simulink model "SSi_liftup"  (R2024b)
settings: Solver=ode1  StartTime=0.0  StopTime=20  FixedStep=0.002  RelTol=1e-3  EnableMultiTasking=on
PostLoadFcn:
  | qc_set_target_type(getConfigSet(bdroot, 'QUARC Default Target Configuration'));
undefined symbols (not defined in the file): A_sw, Aobs, Aobs_d, B_sw, Bobs, Bobs_d, c_star, C_sw, Cobs, Cobs_d, DiscIntNeverNeededParam, HIL, init_cond_lift, K5, K_p2, K_phase1_int, K_phase1_pd, P_end, T1_val, t_p1, t_p2, Ts, u_p1, u_p2, ud_neg, ud_pos, V_sat, x_p1, x_p2
libraries: quarc_library x4
settings Model: SimulationMode=external  ExtModeTrigDuration=5000  Creator=pmartin  LastModifiedBy=natha
settings SolverCC: AlgebraicLoopSolver=TrustRegion  PositivePriorityOrder=on
settings DataIOCC: LimitDataPoints=on  SaveFormat=Array  SignalLoggingSaveFormat=ModelDataLogs  ReturnWorkspaceOutputs=off
settings OptimizationCC: ExpressionDepthLimit=2147483647  InitFltsAndDblsToZero=on
settings DebuggingCC: SaveWithParameterizedLinksMsg=none  UnderspecifiedInitializationDetection=Classic  MergeDetectMultiDrivingBlocksExec=none  SolverPrmCheckMsg=warning  MultiTaskDSMMsg=warning  MultiTaskCondExecSysMsg=none  FcnCallInpInsideContextMsg=warning  UnconnectedInputMsg=warning  UnconnectedOutputMsg=warning  UnconnectedLineMsg=warning  StateNameClashWarn=warning  SFUnexpectedBacktrackingDiag=warning  SFNoUnconditionalDefaultTransitionDiag=warning  SFExecutionAtInitializationDiag=none  ArithmeticOperatorsInVariantConditions=warning
settings ModelReferenceCC: PropagateSignalLabelsOutOfModel=off
settings SFSimCC: SimUseLocalCustomCode=off  CustomCodeUndefinedFunction=UseInterfaceOnly
settings RTWCC: RTWUseLocalCustomCode=off  Toolchain=QUARC win64 | nmake (64-bit Windows)  BuildConfiguration=Faster Runs  GPUComputeCapability=3.5
settings CodeAppCC: StateflowObjectComments=on
settings GRTTargetCC: TargetLangStandard=C89/C90 (ANSI)
settings ConfigComp: CovMetricSettings=dw  CovSaveCumulativeToWorkspaceVar=on  CovSaveSingleToWorkspaceVar=on  CovExternalEMLEnable=off

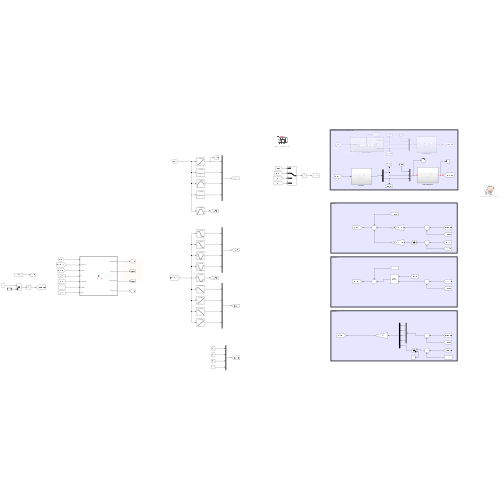
[thumbnail: Simulink's stored preview of the top-level diagram]
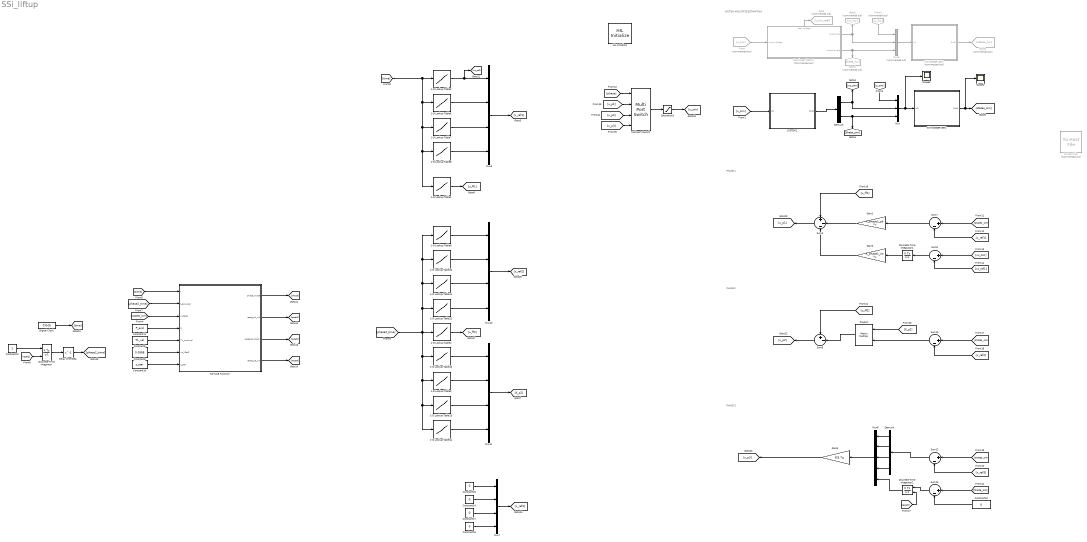
== system SSi_liftup ==
  note: PHASE 1
  note: MOTOR AND STATE ESTIMATION
  note: PHASE 2
  note: PHASE 3
  1-D Lookup Table1 : Lookup_n-D  NumberOfTableDimensions=1  BreakpointsForDimension1=t_p1  Table=u_p1  InternalRulePriority=Speed  RndMeth=Simplest
  1-D Lookup Table10 : Lookup_n-D  NumberOfTableDimensions=1  BreakpointsForDimension1=t_p2  Table=x_p2(:,2)  InternalRulePriority=Speed  RndMeth=Simplest
  1-D Lookup Table11 : Lookup_n-D  NumberOfTableDimensions=1  BreakpointsForDimension1=t_p2  Table=x_p2(:,3)  InternalRulePriority=Speed  RndMeth=Simplest
  1-D Lookup Table12 : Lookup_n-D  NumberOfTableDimensions=1  BreakpointsForDimension1=t_p2  Table=x_p2(:,4)  InternalRulePriority=Speed  RndMeth=Simplest
  1-D Lookup Table13 : Lookup_n-D  NumberOfTableDimensions=1  BreakpointsForDimension1=t_p2  Table=K_p2(:,3)  InternalRulePriority=Speed  RndMeth=Simplest
  1-D Lookup Table14 : Lookup_n-D  NumberOfTableDimensions=1  BreakpointsForDimension1=t_p2  Table=K_p2(:,4)  InternalRulePriority=Speed  RndMeth=Simplest
  1-D Lookup Table15 : Lookup_n-D  NumberOfTableDimensions=1  BreakpointsForDimension1=t_p2  Table=K_p2(:,1)  InternalRulePriority=Speed  RndMeth=Simplest
  1-D Lookup Table2 : Lookup_n-D  NumberOfTableDimensions=1  BreakpointsForDimension1=t_p1  Table=x_p1(:,1)  InternalRulePriority=Speed  RndMeth=Simplest
  1-D Lookup Table3 : Lookup_n-D  NumberOfTableDimensions=1  BreakpointsForDimension1=t_p2  Table=K_p2(:,2)  InternalRulePriority=Speed  RndMeth=Simplest
  1-D Lookup Table4 : Lookup_n-D  NumberOfTableDimensions=1  BreakpointsForDimension1=t_p2  Table=u_p2  InternalRulePriority=Speed  RndMeth=Simplest
  1-D Lookup Table6 : Lookup_n-D  NumberOfTableDimensions=1  BreakpointsForDimension1=t_p1  Table=x_p1(:,2)  InternalRulePriority=Speed  RndMeth=Simplest
  1-D Lookup Table7 : Lookup_n-D  NumberOfTableDimensions=1  BreakpointsForDimension1=t_p1  Table=x_p1(:,3)  InternalRulePriority=Speed  RndMeth=Simplest
  1-D Lookup Table8 : Lookup_n-D  NumberOfTableDimensions=1  BreakpointsForDimension1=t_p1  Table=x_p1(:,4)  InternalRulePriority=Speed  RndMeth=Simplest
  1-D Lookup Table9 : Lookup_n-D  NumberOfTableDimensions=1  BreakpointsForDimension1=t_p2  Table=x_p2(:,1)  InternalRulePriority=Speed  RndMeth=Simplest
  Constant10 : Constant  Value=c_star
  Constant11 : Constant  Value=P_end
  Constant12 : Constant
  Constant{13..17} (5 alike) : Constant  Value=0
  Constant8 : Constant  Value=T1_val
  Constant9 : Constant  Value=0.0568
  Delay One Step : Delay  DelayLength=1
  Demux3 : Demux  Outputs=2
  Demux4 : Demux
  Digital Clock : DigitalClock  SampleTime=Ts
  Discrete-Time Integrator : DiscreteIntegrator  ExternalReset=rising  SampleTime=-1  ICPrevOutput=DiscIntNeverNeededParam  ICPrevScaledInput=DiscIntNeverNeededParam
  Discrete-Time Integrator1 : DiscreteIntegrator  SampleTime=-1  ICPrevOutput=DiscIntNeverNeededParam  ICPrevScaledInput=DiscIntNeverNeededParam
  Discrete-Time Integrator2 : DiscreteIntegrator  ExternalReset=rising  SampleTime=-1  ICPrevOutput=DiscIntNeverNeededParam  ICPrevScaledInput=DiscIntNeverNeededParam
  From : From  Commented=on  GotoTag=u_hw
  From3 : From  Commented=on  GotoTag=u_hw
  Gain2 : Gain  Gain=K_phase1_pd  Multiplication=Matrix(K*u)
  Gain3 : Gain  Gain=K_phase1_int  Multiplication=Matrix(K*u)
  Gain5 : Gain  Gain=K5  Multiplication=Matrix(K*u)
  Goto : Goto  Commented=on  GotoTag=u_hw_real
  Goto1 : Goto  Commented=on  GotoTag=theta_hw
  Goto2 : Goto  Commented=on  GotoTag=xc_hw
  Goto8 : Goto  Commented=on  GotoTag=states_hw
  HIL Initialize : quarc_library/Data Acquisition/Generic/Configuration/HIL Initialize  object_name=HIL-1  board_type=---- Quanser ----  board_number=0  board_options=d0=digital;d1=digital;led=auto;update_rate=normal  exclusive=off  active=off  hardware_clocks=[0:2]  clock_modes=[]  initial_clock_frequencies=[]  set_clock_params_at_start=off  set_clock_params_at_switch_in=off  set_clock_frequencies_at_start=off  set_clock_frequencies_at_switch_in=off  analog_input_channels=[0:1]  analog_input_configurations=[]  analog_input_maximums=10  analog_input_minimums=-10  set_analog_input_params_at_start=on  set_analog_input_params_at_switch_in=off  analog_output_channels=[0:1]  analog_output_maximums=10  analog_output_minimums=-10  initial_analog_outputs=[0]  final_analog_outputs=[0]  watchdog_analog_outputs=0  set_analog_output_params_at_start=on  set_analog_output_params_at_switch_in=off  set_analog_outputs_at_start=on  set_analog_outputs_at_switch_in=off  set_analog_outputs_at_terminate=on  set_analog_outputs_at_switch_out=off  set_analog_outputs_on_watchdog=off  digital_input_channels=[]  digital_output_channels=[0:7]  digital_output_configuration=[]  initial_digital_outputs=[0]  final_digital_outputs=[0]  watchdog_digital_outputs=[0]  set_digital_output_params_at_start=off  set_digital_output_params_at_switch_in=off  set_digital_outputs_at_start=on  set_digital_outputs_at_switch_in=off  set_digital_outputs_at_terminate=on  set_digital_outputs_at_switch_out=off  set_digital_outputs_on_watchdog=off  encoder_channels=[0:1]  quadrature=[4]  encoder_filter_frequency=[]  initial_encoder_counts=[0]  set_encoder_params_at_start=on  set_encoder_params_at_switch_in=off  set_encoder_counts_at_start=on  set_encoder_counts_at_switch_in=off  pwm_channels=[]  pwm_modes=[0]  pwm_frequency=1/0.020  pwm_configuration=[]  pwm_alignment=[]  pwm_polarity=[]  pwm_leading_deadband=[]  pwm_trailing_deadband=[]  initial_pwm_outputs=[0]  final_pwm_outputs=[0]  watchdog_pwm_outputs=[0]  set_pwm_params_at_start=on  set_pwm_params_at_switch_in=off  set_pwm_outputs_at_start=on  set_pwm_outputs_at_switch_in=off  set_pwm_outputs_at_terminate=on  set_pwm_outputs_at_switch_out=off  set_pwm_outputs_on_watchdog=off  other_output_channels=[]  initial_other_outputs=[]  final_other_outputs=[]  watchdog_other_outputs=[]  set_other_outputs_at_start=off  set_other_outputs_at_switch_in=off  set_other_outputs_at_terminate=off  set_other_outputs_at_switch_out=off  set_other_outputs_on_watchdog=off
  HW OBSERVER1 : Subsystem  Commented=on
  MATLAB Function : MATLAB Function  TreatAsAtomicUnit=on
  Multiport Switch : MultiPortSwitch  SaturateOnIntegerOverflow=off  InputSameDT=off
  Mux : Mux  Inputs=3
  Mux{7,9..11} (4 alike) : Mux
  Mux6 : Mux  Commented=on  Inputs=3
  Mux8 : Mux  Inputs=5
  Non-linear Motor1 : Subsystem  Commented=on
      settings: PortSchema="{\"entries\":[{\"content\":{\"sides\":[{\"content\":{\"connectorIds\":[\"In1\"]},\"type\":\"ConnectorPlacement.EquallySpacedRectSide\",\"uuid\":\"8ae262a2-80f5-49ad-9b79-cc35ec5329ff\"},{\"content\":{\"connectorIds\":[\"Out1\",\"Out2\"],\"side\":\"RIGHT\"},\"type\":\"ConnectorPlacement.EquallySpacedRectSide\",\"uuid\":\"cff0d77c-9ae7-4fa2-97d7-b58b6cdbe1a2\"},{\"content\":{\"connectorIds\":[\"Out3\"],\"side\":\"TOP\"},\"type\":\"ConnectorPlacement.EquallySpacedRectSide\",\"uuid\":\"5d4527f6-0b4e-4e3d-a127-4f94b563ffba\"}]},\"type\":\"ConnectorPlacement.EquallySpacedConnector\",\"uuid\":\"e038adc8-37ae-49b9-ae92-fde38d51b088\"}],\"packageUris\":[\"http://schema.mathworks.com/mf0/Connector/R2020b\"],\"version\":\"1.0\"}"
  Product : Product  Multiplication=Matrix(*)
  SYM OBSERVER1 : Subsystem
  SYSTEM1 : Subsystem
  Saturation2 : Saturate  UpperLimit=6  LowerLimit=-6
  Scope2 : Scope
  Scope3 : Scope
  Sum{7..8,10,12..13} (5 alike) : Sum  Inputs=|+-
  Sum3 : Sum  Inputs=+--
  Sum9 : Sum  Inputs=+-|
  To Host File : quarc_library/Sinks/To Host/To Host File  Commented=on  source=Specify via dialog (do not evaluate)  file_name=data_%{date}_%{time}.mat  variable_name=data  decimation=1  sample_time=-1  file_format=MAT-file v.4  options=No header or footer  append=off  final_file_name=data_22-May-2026_21-27-47.mat  encoding=Default  bitrate=0
  wires:
  From/1 -> Non-linear Motor1/1(input voltage)
  [u_sim] -> SYSTEM1/1(In1)
  SYSTEM1/1(Out1) -> Demux3/1
  Non-linear Motor1/3(real voltage) -> Goto/1
  Demux3/1 -> Mux/2, [xc_sim]
  Demux3/2 -> [theta_sim], Mux/3
  Constant8/1 -> MATLAB Function/5(T1_nominal)
  Constant9/1 -> MATLAB Function/6(xc_liftoff)
  Constant10/1 -> MATLAB Function/7(c_star)
  [u_sim] -> Mux/1
  Mux/1 -> Scope3/1, SYM OBSERVER1/1(In1)
  From3/1 -> Mux6/1
  Non-linear Motor1/1(output pos) -> Mux6/2, Goto2/1
  Mux6/1 -> HW OBSERVER1/1(In1)
  Non-linear Motor1/2(output angle) -> Mux6/3, Goto1/1
  HW OBSERVER1/1(Out1) -> Goto8/1
  SYM OBSERVER1/1(Out1) -> Scope2/1, [states_sim]
  [time] -> MATLAB Function/1(t)
  Constant11/1 -> MATLAB Function/4(P)
  Digital Clock/1 -> [time]
  [states_sim] -> MATLAB Function/3(x_state)
  MATLAB Function/1(phase_mode) -> [phase]
  MATLAB Function/2(reset_p1_int) -> [reset1]
  MATLAB Function/3(reset_p2_clock) -> [reset2]
  MATLAB Function/4(reset_p3_int) -> [reset3]
  Constant12/1 -> Discrete-Time Integrator/1
  Discrete-Time Integrator/1 -> Delay One Step/1
  [reset2] -> Discrete-Time Integrator/2
  [phase2_time] -> MATLAB Function/2(t_p2_local)
  1-D Lookup Table1/1 -> [u_ff1]
  1-D Lookup Table4/1 -> [u_ff2]
  [phase] -> Multiport Switch/1
  Multiport Switch/1 -> Saturation2/1
  Sum3/1 -> [u_p1]
  [states_sim] -> Sum7/1
  [x_ref1] -> Sum7/2
  [xc_sim] -> Sum8/1
  [xc_ref1] -> Sum8/2
  Sum8/1 -> Discrete-Time Integrator1/1
  Sum7/1 -> Gain2/1
  Discrete-Time Integrator1/1 -> Gain3/1
  [u_ff1] -> Sum3/1
  Gain2/1 -> Sum3/2
  Gain3/1 -> Sum3/3
  [u_p1] -> Multiport Switch/2
  [u_ff2] -> Sum9/1
  Product/1 -> Sum9/2
  Sum9/1 -> [u_p2]
  Sum10/1 -> Product/2
  [states_sim] -> Sum10/1
  [x_ref2] -> Sum10/2
  Constant13/1 -> Sum13/2
  Gain5/1 -> [u_p3]
  [theta_sim] -> Sum13/1
  Sum13/1 -> Discrete-Time Integrator2/1
  Discrete-Time Integrator2/1 -> Mux8/5
  [states_sim] -> Sum12/1
  [x_ref3] -> Sum12/2
  Constant17/1 -> Mux7/3
  Constant15/1 -> Mux7/1
  Constant16/1 -> Mux7/4
  Constant14/1 -> Mux7/2
  Mux7/1 -> [x_ref3]
  [u_p2] -> Multiport Switch/3
  [u_p3] -> Multiport Switch/4
  Sum12/1 -> Demux4/1
  Demux4/1 -> Mux8/1
  Demux4/2 -> Mux8/2
  Demux4/3 -> Mux8/3
  Demux4/4 -> Mux8/4
  Mux8/1 -> Gain5/1
  [K_p2] -> Product/1
  [reset3] -> Discrete-Time Integrator2/2
  [time] -> 1-D Lookup Table2/1, 1-D Lookup Table6/1, 1-D Lookup Table8/1, 1-D Lookup Table1/1, 1-D Lookup Table7/1
  1-D Lookup Table2/1 -> [xc_ref1], Mux9/1
  1-D Lookup Table6/1 -> Mux9/2
  1-D Lookup Table7/1 -> Mux9/3
  1-D Lookup Table8/1 -> Mux9/4
  Mux9/1 -> [x_ref1]
  1-D Lookup Table11/1 -> Mux10/3
  1-D Lookup Table10/1 -> Mux10/2
  1-D Lookup Table12/1 -> Mux10/4
  1-D Lookup Table9/1 -> Mux10/1
  Mux10/1 -> [x_ref2]
  [phase2_time] -> 1-D Lookup Table14/1, 1-D Lookup Table13/1, 1-D Lookup Table3/1, 1-D Lookup Table15/1, 1-D Lookup Table12/1, 1-D Lookup Table11/1, 1-D Lookup Table10/1, 1-D Lookup Table9/1, 1-D Lookup Table4/1
  1-D Lookup Table13/1 -> Mux11/3
  1-D Lookup Table3/1 -> Mux11/2
  1-D Lookup Table15/1 -> Mux11/1
  Mux11/1 -> [K_p2]
  1-D Lookup Table14/1 -> Mux11/4
  Delay One Step/1 -> [phase2_time]
  Saturation2/1 -> [u_sim]

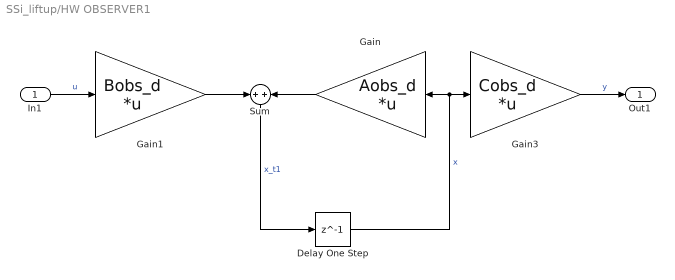
== system SSi_liftup/HW OBSERVER1 ==
  In1 : Inport
  Delay One Step : Delay  DelayLength=1
  Gain : Gain  Gain=Aobs_d  Multiplication=Matrix(K*u)
  Gain1 : Gain  Gain=Bobs_d  Multiplication=Matrix(K*u)
  Gain3 : Gain  Gain=Cobs_d  Multiplication=Matrix(K*u)
  Sum : Sum
  Out1 : Outport
  wires:
  In1/1 -> Gain1/1  "u"
  Gain/1 -> Sum/2
  Gain1/1 -> Sum/1
  Delay One Step/1 -> Gain3/1, Gain/1  "x"
  Sum/1 -> Delay One Step/1  "x_t1"
  Gain3/1 -> Out1/1  "y"

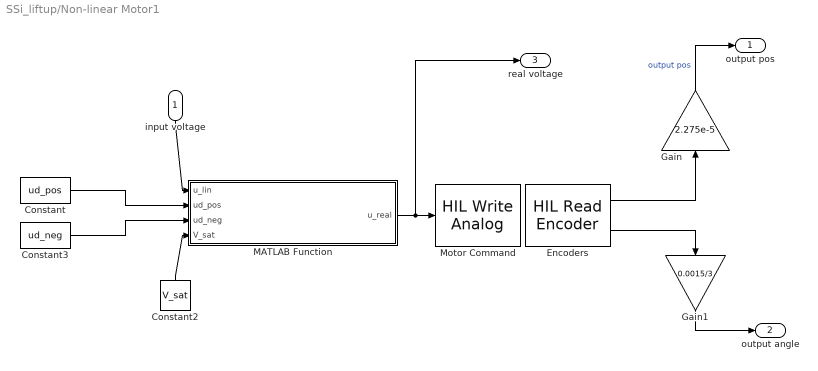
== system SSi_liftup/Non-linear Motor1 ==
  input voltage : Inport
  Constant : Constant  Value=ud_pos
  Constant2 : Constant  Value=V_sat
  Constant3 : Constant  Value=ud_neg
  Encoders : quarc_library/Data Acquisition/Generic/Immediate I//O/HIL Read Encoder  object_name=HIL-1  channels=[0,1]  sample_time=qc_get_step_size  active=on  vector_output=off  data_type_mode=Inherit via back propagation  data_type=double
  Gain : Gain  Gain=2.275e-5
  Gain1 : Gain  Gain=0.0015/3
  MATLAB Function : MATLAB Function  TreatAsAtomicUnit=on
  Motor Command : quarc_library/Data Acquisition/Generic/Immediate I//O/HIL Write Analog  object_name=HIL-1  channels=0  sample_time=-1  active=off  vector_input=off
  output pos : Outport
  output angle : Outport  Port=2
  real voltage : Outport  Port=3
  wires:
  Encoders/1 -> Gain/1
  input voltage/1 -> MATLAB Function/1(u_lin)
  Gain/1 -> output pos/1  "output pos"
  MATLAB Function/1(u_real) -> real voltage/1, Motor Command/1
  Constant/1 -> MATLAB Function/2(ud_pos)
  Constant3/1 -> MATLAB Function/3(ud_neg)
  Constant2/1 -> MATLAB Function/4(V_sat)
  Encoders/2 -> Gain1/1
  Gain1/1 -> output angle/1

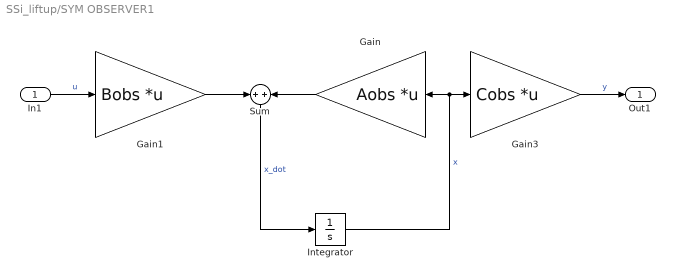
== system SSi_liftup/SYM OBSERVER1 ==
  In1 : Inport
  Gain : Gain  Gain=Aobs  Multiplication=Matrix(K*u)
  Gain1 : Gain  Gain=Bobs  Multiplication=Matrix(K*u)
  Gain3 : Gain  Gain=Cobs  Multiplication=Matrix(K*u)
  Integrator : Integrator  InitialCondition=init_cond_lift  LimitOutput=on  UpperSaturationLimit=[0.407, deg2rad(11.66), inf, inf]  LowerSaturationLimit=-[0.407, deg2rad(11.66), inf, inf]
  Sum : Sum
  Out1 : Outport
  wires:
  In1/1 -> Gain1/1  "u"
  Gain/1 -> Sum/2
  Gain1/1 -> Sum/1
  Integrator/1 -> Gain3/1, Gain/1  "x"
  Sum/1 -> Integrator/1  "x_dot"
  Gain3/1 -> Out1/1  "y"

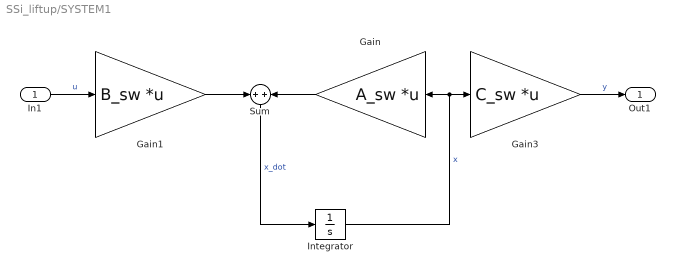
== system SSi_liftup/SYSTEM1 ==
  In1 : Inport
  Gain : Gain  Gain=A_sw  Multiplication=Matrix(K*u)
  Gain1 : Gain  Gain=B_sw  Multiplication=Matrix(K*u)
  Gain3 : Gain  Gain=C_sw  Multiplication=Matrix(K*u)
  Integrator : Integrator  InitialCondition=init_cond_lift  LimitOutput=on  UpperSaturationLimit=[0.407, deg2rad(11.66), inf, inf]  LowerSaturationLimit=-[0.407, deg2rad(11.66), inf, inf]
  Sum : Sum
  Out1 : Outport
  wires:
  In1/1 -> Gain1/1  "u"
  Gain/1 -> Sum/2
  Gain1/1 -> Sum/1
  Integrator/1 -> Gain3/1, Gain/1  "x"
  Sum/1 -> Integrator/1  "x_dot"
  Gain3/1 -> Out1/1  "y"

== matlab function SSi_liftup/Non-linear Motor1/MATLAB Function ==
  data: u_lin input; u_real output; ud_pos input; ud_neg input; V_sat input
function u_real = non_linear_deadzone(u_lin, ud_pos, ud_neg, V_sat)

epsilon = 0.1;

if u_lin > epsilon
    u_real = u_lin + ud_pos;
    
elseif u_lin < -epsilon
    u_real = u_lin - ud_neg;
    
else
    u_real = 0;
end

if u_real > V_sat
    u_real = V_sat;
elseif u_real < -V_sat
    u_real = -V_sat;
end

== matlab function SSi_liftup/MATLAB Function ==
  settings: updateMethod=DISCRETE
  data: t input; t_p2_local input; phase_mode output; x_state input; P input; reset_p1_int output; reset_p2_clock output; reset_p3_int output; T1_nominal input; xc_liftoff input; c_star input
function [phase_mode, reset_p1_int, reset_p2_clock, reset_p3_int] = phase_manager(t, t_p2_local, x_state, P, T1_nominal, xc_liftoff, c_star)

    
    % Persistent memory ensures the state machine only moves forward
    persistent current_phase;
    
    if isempty(current_phase)
        current_phase = 1;
    end
    
    % 1. Force the input into a strict column vector
    x_col = x_state(:);
    
    % 2. Extract cart position
    xc = x_col(1);
    
    % 3. Compute Lyapunov Matrix [1x1]
    V_matrix = x_col' * P * x_col;
    
    % 4. Force to pure scalar to prevent C-coder logical errors!
    V = V_matrix(1);       
    c_scalar = c_star(1);  % Safeguard c_star as well

    % =========================================================
    % STATE TRANSITION LOGIC
    % =========================================================
    
    % --- Transition 1 -> 2 (Table Approach -> Swing Up) ---
    % Trigger if we reach the nominal time AND we are within 1mm of the lift-off position.
    if current_phase == 1 && t >= T1_nominal && xc >= (xc_liftoff - 0.001)
        current_phase = 2;
    end
    
    % --- Transition 2 -> 3 (Swing Up -> RoA Catch) ---
    % Wait until we are at least 0.5s into the local Phase 2 swing-up 
    % (to prevent accidental early triggers), then check the Lyapunov boundary.
    if current_phase == 2 && t_p2_local > 0.5 && V <= c_scalar
        current_phase = 3;
    end
    
    % =========================================================
    % SIGNAL OUTPUTS
    % =========================================================
    
    phase_mode = current_phase;
    
    % 1. Phase 1 Cart Integrator Reset
    if current_phase == 1
        reset_p1_int = false; % Allow integration during approach
    else
        reset_p1_int = true;  % Kill it the exact millisecond Phase 2 starts
    end
    
    % 2. Phase 2 Local Stopwatch Reset
    if current_phase == 1
        reset_p2_clock = true; % Hold the stopwatch at exactly 0.00s
    else
        reset_p2_clock = false; % Release it! It will now count up seamlessly.
    end
    
    % 3. Phase 3 Angle Integrator Reset
    if current_phase == 3
        reset_p3_int = false; % Release it to lock onto the vertical equilibrium
    else
        reset_p3_int = true;  % Keep it dead during Phase 1 and 2 to prevent wind-up
    end
    
end
